simulink model "RB_KAIROS_BaseOnly"  (R2020b)
settings: Solver=ode4  StartTime=0.0  StopTime=t_end  FixedStep=Ts  RelTol=1e-3
values from neighbouring files (symbols this model uses):
  am = 0.3    [RB_KAIROS_ImpControl_OpSpace_BaseOnly.m]
  am_r = 0.3    [RB_KAIROS_ImpControl_OpSpace_BaseOnly.m]
  Jv = [1 0 0; 0 1 0; 0 0 0; 0 0 0; 0 0 0; 0 0 1;]    [RB_KAIROS_ImpControl_OpSpace_BaseOnly.m]
  Kc = diag(5*[1000,1000,0,0,0,1000])    [RB_KAIROS_ImpControl_OpSpace_BaseOnly.m]
  model_sample_time = 0.001    [RB_KAIROS_ImpControl_OpSpace_BaseOnly.m]
  q_dot_0 = zeros(10,1)    [RB_KAIROS_ImpControl_OpSpace_BaseOnly.m]
  T_i = T_W_V    [RB_KAIROS_ImpControl_OpSpace_BaseOnly.m]
  tau_ext = [0 0 0]    [RB_KAIROS_ImpControl_OpSpace_BaseOnly.m]
  v_SMU = 10    [RB_KAIROS_ImpControl_OpSpace_BaseOnly.m]
  vm = 0.6    [RB_KAIROS_ImpControl_OpSpace_BaseOnly.m]
  vm_r = 0.6    [RB_KAIROS_ImpControl_OpSpace_BaseOnly.m]
undefined symbols (not defined in the file or in its folder): DiscIntNeverNeededParam, magnitude, q_0, T_f
libraries: simulink x4, utils x4, transformations_lib x1
(part 16 of 16)

== matlab function RB_KAIROS_BaseOnly/Trajectory Generator/move2pose/MATLAB Function ==
  data: in input; reset input; out output
function out = fcn(in,reset)
%%% This is kind of a Memory block for one boolean.
% output is equal input as long as input is not zero.
% If input becomes zero, output STAYS zero, till reset is triggered.


persistent memory 
if isempty(memory)
    memory = 0;       %remembers the state
end

out = in;

if in == 0
    memory = 1;
end

if memory == 1
    out = 0;
    if reset>0
        memory = 0;
    end
end

end

== matlab function RB_KAIROS_BaseOnly/Trajectory Generator/Subsystem1/Angle Axis Via Quaternions/r2q ==
  data: R input; q output
function q =r2q(R)
%#codegen
q=zeros(1,4);
if ~(all(size(R)==[3,3]))
    error('Bad input dimensions. Input must be 3x3');
end

% Ne dela za specialne kote, ko je s=0 ali v=0
% s=0.5*sqrt(R(1,1)+R(2,2)+R(3,3)+1);
% v=[R(3,2)-R(2,3),R(1,3)-R(3,1),R(2,1)-R(1,2)]'/4/s;
%
% q=quaternion([s v']);

qsx=trace(R)+1;
if qsx>=0
    qs = sqrt(qsx)/2.0;
else
    qs=0;
end
kx = R(3,2) - R(2,3);	% Oz - Ay
ky = R(1,3) - R(3,1);	% Ax - Nz
kz = R(2,1) - R(1,2);	% Ny - Ox

if (R(1,1) >= R(2,2)) && (R(1,1) >= R(3,3))
    kx1 = R(1,1) - R(2,2) - R(3,3) + 1;	% Nx - Oy - Az + 1
    ky1 = R(2,1) + R(1,2);			% Ny + Ox
    kz1 = R(3,1) + R(1,3);			% Nz + Ax
    add = (kx >= 0);
elseif (R(2,2) >= R(3,3))
    kx1 = R(2,1) + R(1,2);			% Ny + Ox
    ky1 = R(2,2) - R(1,1) - R(3,3) + 1;	% Oy - Nx - Az + 1
    kz1 = R(3,2) + R(2,3);			% Oz + Ay
    add = (ky >= 0);
else
    kx1 = R(3,1) + R(1,3);			% Nz + Ax
    ky1 = R(3,2) + R(2,3);			% Oz + Ay
    kz1 = R(3,3) - R(1,1) - R(2,2) + 1;	% Az - Nx - Oy + 1
    add = (kz >= 0);
end

if add
    kx = kx + kx1;
    ky = ky + ky1;
    kz = kz + kz1;
else
    kx = kx - kx1;
    ky = ky - ky1;
    kz = kz - kz1;
end
nm = norm([kx ky kz]);
if nm == 0
    q = [1 0 0 0];
else
    ss=1-qs^2;
    if ss<0
        s=0;
    else
        s = sqrt(ss) / nm;
    end
    qv = s*[kx ky kz];
    
    q = [qs qv];
end

== matlab function RB_KAIROS_BaseOnly/Trajectory Generator/move2pose/Multicall ==
  data: human_dist input; human output; crit1 input; crit2 input; crit3 input; n_steps input; v_SMU input; v_SMU_step output; v_max input; v_human input; Tm output; v_human_opt input
function [human,v_SMU_step,Tm] = Multicall(human_dist,crit1,crit2,crit3,n_steps,v_SMU,v_max,v_human,v_human_opt)
% MULTICALL is a block which introduces several velocity levels between the
% maximum velocity and the safe velocity. Therefore it calls the adaption
% function multiple times with intermediate velocities. It has also a
% hysteresis, that means if the human leaves a region it is not directly
% the higher velocity applied. Only if the human leaves the next region the
% velocity rises again. 
% 
% The crit values determine the distances when to shift: 
% crit1 is the distance nearest to the robot, so here is v_SMU applied.
% crit2 is the distance when a human enters there, the velocity starts to
% decline
% crit3 is the largest distance since it is the hysteresis level for crit2,
% this means if the human distance is greater than crit3 the v_max is
% applied. 
% crit1 OR crit2 OR crit3 can be set to -1, then it is calculated
% automatically like:
% crit1 = crit2-crit_step*n_steps (crit_step = crit3-crit2)
% crit2 = crit3-crit_step
% crit3 = crit2+crit_step
%
% n_steps determines how many intermediate velocity levels should be
% applied, so n_steps=0 means deactivation of the intermediate levels.
% All distances are assumed to be positive values.

% Inputs:
% human_dist    current distance human-robot in meters
% crit1         nearest critical distance to robot
% crit2         level when to activate decline
% crit3         farest level to robot (deactivate all)
% n_steps       number of intermediate velocity levels
% v_SMU         low safe velocity
% v_max         high maximum velocity
% v_human       velocity of human for calc Tm, negative value means human
%               is approaching robot, positive value means human is leaving
%               If no real data is available an always positive estimate
%               can also be set here, see also next input.
% v_human_opt   Boolean; Set to 1 if v_human is real data, means with sign.
%               Set to 0 if v_human is always positive estimate, the sign
%               is estimated then from the human_distance. Actually it is
%               safe against wrong settings, except one special case: If
%               the human_dist data is noisy and the difference between two
%               measurements would indicate a negative velocity, but
%               actually the velocity is still positive. In this case the
%               code sets a negative velocity, if you don't set v_human_opt
%               to true.

% Outputs:
% human         boolean; True if human is near
% v_SMU_step    current desired velocity level
% Tm            time duration till when the adaption has to be completed

%n_steps in the code means in how many steps one adapts the velocity (so at least 1)
n_steps = n_steps+1; 

% Calculate the step sizes in distance ...
if crit1<0 % If crit1 is auto set
    crit_step = crit3-crit2;
    crit1 = crit2-crit_step*n_steps; %Assumption for crit1
elseif crit2<0 % If crit2 is auto set
    crit_step = (crit3-crit1)/(n_steps+1);
    crit2 = crit3-crit_step; %Assumption for crit2
elseif crit3<0 % If crit3 is auto set
    crit_step = (crit2-crit1)/n_steps;
    crit3 = crit2+crit_step; %Assumption for crit3
else
    crit_step = (crit2-crit1)/n_steps;
end
% ... and velocity
v_step = (v_max-v_SMU)/n_steps;

persistent human_1 v_SMU_step_1 human_trigger human_dist_1 %last_trigger 
if isempty(human_1)  %remembers the human state from last run
    if human_dist<=crit2 %only init
        human_1 = 1;
    else
        human_1 = 0;
    end
end
if isempty(v_SMU_step_1)   %remembers the v_SMU_step from last run
    if human_dist<=crit2 %only init
        v_SMU_step_1 = v_SMU;
    else
        v_SMU_step_1 = v_max; 
    end
end
if isempty(human_trigger)
    human_trigger = 0;    %remembers the human_trigger, so which border is triggered
end
if isempty(human_dist_1)
    human_dist_1 = human_dist;    %remembers the human_distance from last run, to auto calc sign(v_human)
end

% if v_human is an estimate without sign the sign is estimated from two
% human_distances, but this might cause errors, due to noise in human_dist.
% Thats why the option is still there. But if someone sends real data
% (especially negative values) and forgets to set option true, this would
% also cause problems, therefore if v_human is negative it is not again
% multiplied (what would make it positive!)
if v_human_opt == false && v_human>0
    v_human = v_human*sign(human_dist-human_dist_1);
end

% First set old values, if no changes occur
human = human_1;
v_SMU_step = v_SMU_step_1;

% compute borders
borders = zeros(n_steps+1,1);
for i=0:n_steps
   borders(i+1) = crit2-i*crit_step; %compute distance borders between crit1 and crit2 (inclusive both)
end

borders2 = borders+ones(size(borders))*crit_step; %shift to crit3
borders2(1) = crit3; %override for crit3, if crit3~=Assumption
region = xor(borders<human_dist,borders2<human_dist); %region is a vector with a single 1 at that region in which the human is currently
[region_max,ind] = max(region); %search for index of region

if region_max==0 %But if no 1 is contained in region, the human is somewhere else
    if human_dist>crit3 %human far away
        ind = 0;
    elseif human_dist<=crit1 %human very close
        ind = n_steps+1;
    end
end

% Slow down transition 
if ind>=2 && human_trigger<ind-1 %if human is at least in second region and this region is not triggered jet
    human = 1; % activate human bit
    human_trigger = ind-1;
    
% Speed up transition
elseif ind<=n_steps-1 && human_trigger>ind %if human is at least two steps away from robot and this region was triggered somewhen
    if ind==0 %if human is far away; switch adaption of
        human = 0;
        v_SMU_step = v_max;
    else
        human = 1;
    end
    human_trigger = ind;
end

%calculate new velocity, for the current triggered border
v_SMU_step = v_max - v_step*human_trigger; 

% Calc Tm
inf_time = 10000;
if human_dist<=crit1 %human very close => No time for adaption left
    Tm = 0;
elseif human_dist>crit3 %human very far => inf time for adaption left
    Tm = inf_time;
else
    if abs(v_human)<=1e-4 %human is nearly standing still => inf time to adapt
        Tm = inf_time;
    elseif v_human>0 %human is leaving => inf time to adapt
        Tm = inf_time;
    else
        if human_trigger==0
            crit_th = borders(2); %outside crit2 the nearest border for adapt is the next nearer border seen from crit2
        else
            crit_th = borders(human_trigger+1); %in general set crit threshold to next nearer border
        end
        % abs(v) because velocity is negative here
        Tm = (human_dist-crit_th)/abs(v_human); 
        
    end
end

% remeber current settings
human_1 = human;
v_SMU_step_1 = v_SMU_step;
human_dist_1 = human_dist;

end %end of function

%% Two steps version
% % Sequence of ifs is important, if greater steps occur!!
% % Slow down transitions
% if human_dist < crit2-crit_step*2 && human_trigger(3) == 0
%     v_SMU_step = v_max - v_step*3;
%     human = 1;
%     human_trigger(3) = 1;
%     human_trigger(2) = 1;
%     human_trigger(1) = 1;
% elseif human_dist < crit2-crit_step && human_trigger(2) == 0
%     v_SMU_step = v_max - v_step*2;
%     human = 1;
%     human_trigger(2) = 1;
%     human_trigger(1) = 1;
% elseif human_dist < crit2 && human_trigger(1) == 0
%     v_SMU_step = v_max - v_step;
%     human = 1;
%     human_trigger(1) = 1;
%     
% % Speed up transitions
% elseif human_dist > crit3 && human_trigger(1) == 1
%     v_SMU_step = v_max;
%     human = 0;
%     human_trigger(1) = 0; 
%     human_trigger(2) = 0;
%     human_trigger(3) = 0;
% elseif human_dist > crit2 && human_trigger(2) == 1
%     v_SMU_step = v_max - v_step;
%     human = 1;
%     human_trigger(2) = 0;
%     human_trigger(3) = 0;  
% elseif human_dist > crit2-crit_step && human_trigger(3) == 1 %ind ==2
%     v_SMU_step = v_max - v_step*2;
%     human = 1;
%     human_trigger(3) = 0;
%     
% end


%% Dynamic version; not working
% persistent region_1 human_1 v_SMU_step_1
% if isempty(region_1)
%     region_1 = zeros(n_steps+1,1);    %remembers the psi from last run
% end
% if isempty(human_1)
%     human_1 = 0;    %remembers the psi from last run
% end
% if isempty(v_SMU_step_1)
%     v_SMU_step_1 = v_max;    %remembers the psi from last run
% end
% 
% crit_step = (crit2-crit1)/n_steps;
% crit3 = crit2+crit_step;
% 
% v_step = (v_max-v_SMU)/n_steps;
% 
% region = zeros(n_steps+1,1);
% borders = zeros(n_steps+1,1);
% 
% if human_dist >= crit3 %Human far away
%     human = 0;
%     v_SMU_step = v_SMU;
% elseif human_dist <= crit1 %Human very close
%     human = 1;
%     v_SMU_step = v_SMU;
% else
%     % the complex part inbetween...
%     
%     for i=0:n_steps
%        borders(i+1) = crit2-i*crit_step; %compute distance borders between crit1 and crit2 (inclusive both)
%     end
%     
%     borders2 = borders+ones(size(borders))*crit_step; %shift to crit3
%     region = xor(borders<human_dist,borders2<human_dist); %region is a vector with a single 1 at that region in which the human is currently
%     [~,ind] = max(region);
%     [~,ind_1] = max(region_1);
% 
%     if ind == ind_1 %No change = human in same region
%         human = human_1;
%         v_SMU_step = v_SMU_step_1;
%     elseif ind > ind_1 %steps closer
%         human = 1;
%         v_SMU_step = v_max-v_step;        
%     elseif ind < ind_1 %steps away
%         
%     end
%            
%     
%     
%     region_1 = region;
% end
